simulink library "Drone_MIMO_Simple_Model"  (R2025b)
settings: Solver=VariableStepAuto  StartTime=0.0  StopTime=10.0  RelTol=1e-3
settings Model: Creator=Alek  LastModifiedBy=Alek

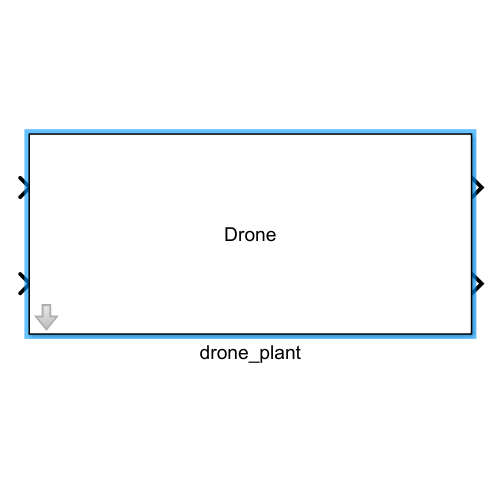
[thumbnail: Simulink's stored preview of the top-level diagram]
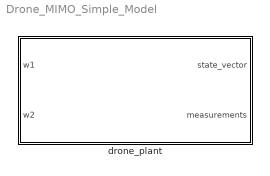
== system Drone_MIMO_Simple_Model ==
  drone_plant : Subsystem  mask{kf=1e-5, m=0.5, l=1e-2, Irod=6.6666e-5}
      mask prompts: kf "Thrust Coefficient"; m "Mass"; l "Arm length"; Irod "Rod Moment Of Intertia"
      mask Display: disp('Drone');

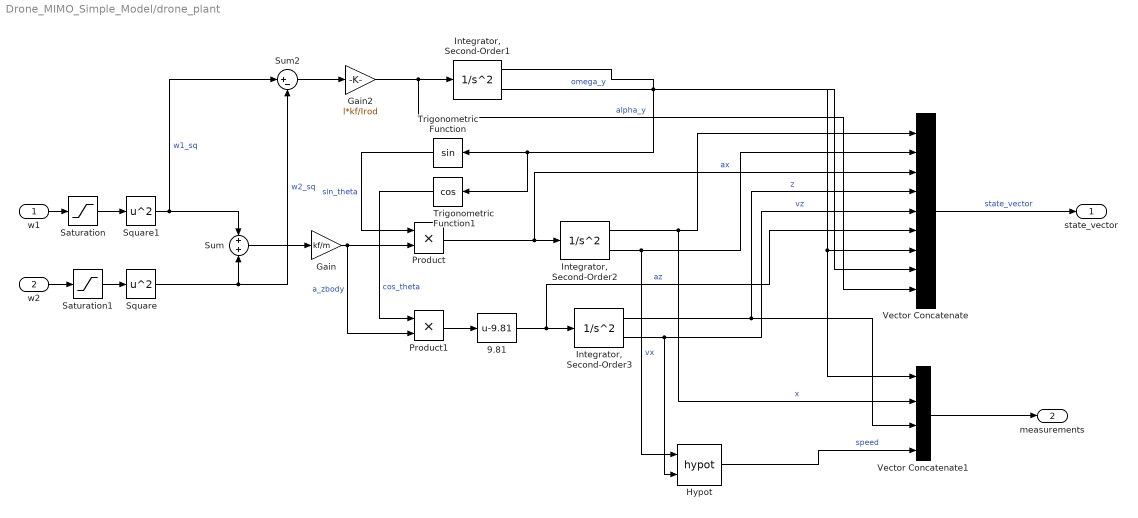
== system Drone_MIMO_Simple_Model/drone_plant ==
  w1 : Inport  OutMin=[0]  PortDimensions=1
  w2 : Inport  Port=2  OutMin=[0]  PortDimensions=1
  9.81 : Bias  Bias=-9.81  SaturateOnIntegerOverflow=off
  Gain : Gain  Gain=kf/m
  Gain2 : Gain  Gain=l*kf/Irod
  Hypot : Math  Operator=hypot
  "Integrator, Second-Order1" : SecondOrderIntegrator
  "Integrator, Second-Order2" : SecondOrderIntegrator  ICX=0
  "Integrator, Second-Order3" : SecondOrderIntegrator  ICX=500  LimitX=on  LowerLimitX=0
  Product : Product
  Product1 : Product
  Saturation : Saturate  UpperLimit=1000  LowerLimit=0
  Saturation1 : Saturate  UpperLimit=1000  LowerLimit=0
  Square : Math  Operator=square
  Square1 : Math  Operator=square
  Sum : Sum  Inputs=+|+
  Sum2 : Sum  Inputs=|+-
  Trigonometric Function : Trigonometry
  Trigonometric Function1 : Trigonometry  Operator=cos
  Vector Concatenate : Concatenate  NumInputs=9
  Vector Concatenate1 : Concatenate  NumInputs=4
  state_vector : Outport
  measurements : Outport  Port=2
  wires:
  Square1/1 -> Sum2/1, Sum/1  "w1_sq"
  9.81/1 -> Vector Concatenate/6, "Integrator, Second-Order3"/1  "az"
  "Integrator, Second-Order1"/1 -> Vector Concatenate1/1, Vector Concatenate/7, Trigonometric Function1/1, Trigonometric Function/1
  "Integrator, Second-Order2"/2 -> Vector Concatenate/2, Hypot/1  "vx"
  Sum/1 -> Gain/1
  Trigonometric Function/1 -> Product/1  "sin_theta"
  Product1/1 -> 9.81/1
  Gain2/1 -> Vector Concatenate/9, "Integrator, Second-Order1"/1  "alpha_y"
  Product/1 -> Vector Concatenate/3, "Integrator, Second-Order2"/1  "ax"
  Square/1 -> Sum2/2, Sum/2  "w2_sq"
  Vector Concatenate1/1 -> measurements/1
  Gain/1 -> Product1/2, Product/2  "a_zbody"
  "Integrator, Second-Order3"/1 -> Vector Concatenate1/3, Vector Concatenate/4  "z"
  Trigonometric Function1/1 -> Product1/1  "cos_theta"
  "Integrator, Second-Order3"/2 -> Hypot/2, Vector Concatenate/5  "vz"
  Hypot/1 -> Vector Concatenate1/4  "speed"
  Sum2/1 -> Gain2/1
  Vector Concatenate/1 -> state_vector/1  "state_vector"
  "Integrator, Second-Order2"/1 -> Vector Concatenate1/2, Vector Concatenate/1  "x"
  "Integrator, Second-Order1"/2 -> Vector Concatenate/8  "omega_y"
  Saturation/1 -> Square1/1
  w1/1 -> Saturation/1
  w2/1 -> Saturation1/1
  Saturation1/1 -> Square/1
